simulink model "MotorXploer"  (R2024b)
settings: Solver=FixedStepAuto  StartTime=0.0  StopTime=inf  FixedStep=0.001  RelTol=1e-3
undefined symbols (not defined in the file or in its folder): Blocking, LF, Non
libraries: hdlsllib x5, amg_usbconverter_n_connect_lib x3
settings Model: Creator=beamk  LastModifiedBy=VICTUS

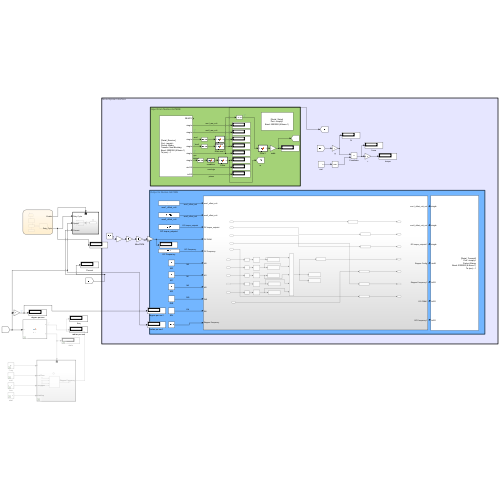
[thumbnail: Simulink's stored preview of the top-level diagram]
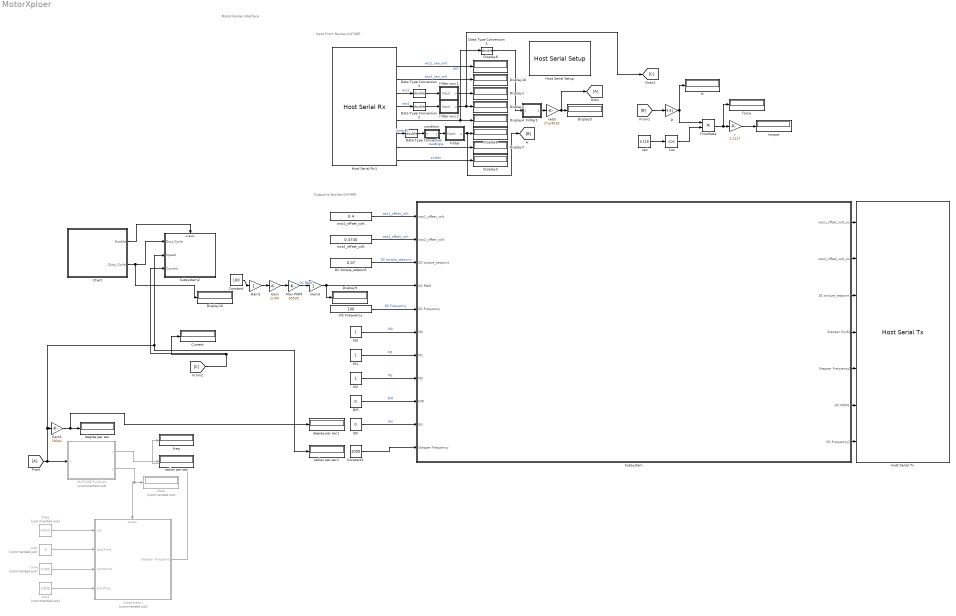
== system MotorXploer ==
  note: Output to Nucleo-G474RE
  note: Input From Nucleo-G474RE
  note: MotorXploler Interface
  Chart : Stateflow chart  TreatAsAtomicUnit=on
      settings: PortSchema="{\"entries\":[{\"content\":{\"sides\":[{\"content\":{},\"type\":\"ConnectorPlacement.EquallySpacedRectSide\",\"uuid\":\"8e28883a-1281-4b20-80f5-117cf80ab28d\"},{\"content\":{\"connectorIds\":[\"Out2\",\"Out1\"],\"side\":\"RIGHT\"},\"type\":\"ConnectorPlacement.EquallySpacedRectSide\",\"uuid\":\"8e6f6195-e9fb-4b08-ac17-6c9691bed55c\"},{\"content\":{\"side\":\"TOP\"},\"type\":\"ConnectorPlacement.EquallySpacedRectSide\",\"uuid\":\"2bfcf31e-5df8-4905-a340-c34624cfbeee\"}]},\"type\":\"ConnectorPlacement.EquallySpacedConnector\",\"uuid\":\"f3782a18-4493-4071-a1dd-9ffba4b12391\"}],\"packageUris\":[\"http://schema.mathworks.com/mf0/Connector/R2020b\"],\"version\":\"1.0\"}"
  Constant : Constant  Value=100
  Constant1 : Constant  Value=1000
  Cos : Trigonometry  Operator=cos
  Current : Display
  DC Frequency : Constant  Value=100
  DC torque_setpoint : Constant  Value=0.07
  DIR : Constant  Value=0  OutDataTypeStr=uint8
  Data Type Conversion{,1..3} (4 alike) : DataTypeConversion  OutDataTypeStr=double  SaturateOnIntegerOverflow=off  RndMeth=Floor
  Display{1..10,16} (11 alike) : Display
  EN : Constant  Value=0  OutDataTypeStr=uint8
  Fcostheta : Product
  Fillter : MATLAB Function  TreatAsAtomicUnit=on
  Fillter1 : MATLAB Function  TreatAsAtomicUnit=on
  Freq : Constant  Commented=on  Value=200000
  From : From
  Gain : Gain  Gain=1/100
  Gain1 : Gain  Gain=180/pi
  Gain2 : Gain
  Gain3 : Gain
  Goto : Goto
  Host Serial Rx1 : amg_usbconverter_n_connect_lib/Host Serial Rx  conf=rx  port=<auto>  baudrate=2000000  databits=8  parity=None  stopbit=1  flowcontrol=None  transfer=Non-Blocking  timeout=5  packetmode=Binary  enableinitialvalues=off  initialvalues=[]  binheader='45'  binterminator='A'  porttype_double=0  porttype_single=6  porttype_int8=0  porttype_uint8=0  porttype_int16=0  porttype_uint16=1  porttype_int32=1  porttype_uint32=0  asciiformat='%f,%f,%d,%d'  rx_asciiterminator="LF (0x0A - \"\\n\")"  tx_asciiterminator="CRLF (0x0D 0x0A - \"\\r\\n\")"  sampletime=-1  enablecustomportlabel=off  cinputportlabel=0  coutputportlabel=A  portpinstr=0  blockid=HostSerialRx1  inputporttype=[]  inputportwidth=[]  inputportlabel={}  outputporttype=[3 1 1 1 1 1 1 5 6]  outputportwidth=[1 1 1 1 1 1 1 1 1]  outputportlabel={'READY','single','single','single','single','single','single','uint16','int32'}  compat=0  optionstring=[]  autoport='<empty>'
  Host Serial Setup : amg_usbconverter_n_connect_lib/Host Serial Setup  conf=setup  port=<auto>  baudrate=2000000  databits=8  parity=None  stopbit=1  flowcontrol=None  transfer=Blocking  timeout=2  packetmode=Binary  initialvalues=[]  binheader='7E 7E'  binterminator='03 03'  porttype_double=0  porttype_single=1  porttype_int8=0  porttype_uint8=0  porttype_int16=0  porttype_uint16=0  porttype_int32=0  porttype_uint32=2  asciiformat='%d %u %x'  rx_asciiterminator="CRLF (0x0D 0x0A - \"\\r\\n\")"  tx_asciiterminator="CRLF (0x0D 0x0A - \"\\r\\n\")"  sampletime=-1  enablecustomportlabel=off  cinputportlabel=0  coutputportlabel=A  portpinstr=0  blockid=HostSerialSetup  inputporttype=[]  inputportwidth=[]  inputportlabel={}  outputporttype=[]  outputportwidth=[]  outputportlabel={}  compat=0  optionstring=[]  autoport='<empty>'
  Host Serial Tx : amg_usbconverter_n_connect_lib/Host Serial Tx  conf=tx  port=<auto>  baudrate=2000000  databits=8  parity=None  stopbit=1  flowcontrol=None  transfer=Blocking  timeout=2  packetmode=Binary  initialvalues=[]  binheader='45'  binterminator='A'  porttype_double=0  porttype_single=3  porttype_int8=0  porttype_uint8=1  porttype_int16=0  porttype_uint16=0  porttype_int32=3  porttype_uint32=0  asciiformat='%d,%f'  rx_asciiterminator="CRLF (0x0D 0x0A - \"\\r\\n\")"  tx_asciiterminator="CRLF (0x0D 0x0A - \"\\r\\n\")"  sampletime=-1  enablecustomportlabel=off  cinputportlabel=0  coutputportlabel=A  portpinstr=0  blockid=HostSerialTx  inputporttype=[1 1 1 3 6 6 6]  inputportwidth=[1 1 1 1 1 1 1]  inputportlabel={'single','single','single','uint8','int32','int32','int32'}  outputporttype=[]  outputportwidth=[]  outputportlabel={}  compat=0  optionstring=[]  autoport='<empty>'
      settings: SourceProductName=aMG USB Converter N
  M0 : Constant  OutDataTypeStr=uint8
  M1 : Constant  OutDataTypeStr=uint8
  M2 : Constant  OutDataTypeStr=uint8
  MATLAB Function : MATLAB Function  Commented=on  TreatAsAtomicUnit=on
  Max PWM : Gain  Gain=65535
  N : Display
  Subsystem : Subsystem
  Subsystem1 : Subsystem  Commented=on
  Subsystem2 : Subsystem
  condition : MATLAB Function  TreatAsAtomicUnit=on
  degree per sec : Display
      settings: Format=decimal (Stored Integer)
  degree per sec1 : Display
      settings: Format=decimal (Stored Integer)
  fillter wcs 1 : MATLAB Function  TreatAsAtomicUnit=on
  fillter wcs 2 : MATLAB Function  TreatAsAtomicUnit=on
  force : Display
  freq : Display
      settings: Format=decimal (Stored Integer)
  g : Gain  Gain=9.81
  r : Gain  Gain=0.1127
  rad : Constant  Value=0.118
  rad/s : Gain  Gain=2*pi/8192
  radian per sec : Display
  radian per sec1 : Display
  start : Constant  Commented=on  Value=1000
  state : Display  Commented=on
  time : Constant  Commented=on  Value=0.003
  torque : Display
  wait : Constant  Commented=on  Value=3
  wcs1_offset_volt : Constant  Value=0.4  OutDataTypeStr=single
  wcs2_offset_volt : Constant  Value=0.4745  OutDataTypeStr=single
  wires:
  Host Serial Rx1/2 -> Display8/1  "wcs1_raw_volt"
  Host Serial Rx1/3 -> Display16/1  "wcs2_raw_volt"
  Host Serial Rx1/7 -> Data Type Conversion/1  "loadcell"
  Host Serial Rx1/5 -> Data Type Conversion2/1  "wcs2"
  Host Serial Rx1/8 -> Display7/1  "rawAngle"
  rad/s/1 -> Goto/1, Display5/1
  Host Serial Rx1/6 -> Data Type Conversion1/1, Display4/1  "pps"
  Host Serial Rx1/4 -> Data Type Conversion3/1  "wcs1"
  Host Serial Rx1/9 -> Display3/1  "pulses"
  wcs1_offset_volt/1 -> Subsystem/1(wcs1_offset_volt)  "wcs1_offset_volt"
  wcs2_offset_volt/1 -> Subsystem/2(wcs2_offset_volt)  "wcs2_offset_volt"
  DC torque_setpoint/1 -> Subsystem/3(DC torque_setpoint)  "DC torque_setpoint"
  Max PWM/1 -> Gain3/1  "DC PWM"
  DC Frequency/1 -> Subsystem/5(DC Frequency)  "DC Frequency"
  M0/1 -> Subsystem/6(M0)  "M0"
  M1/1 -> Subsystem/7(M1)  "M1"
  M2/1 -> Subsystem/8(M2)  "M2"
  DIR/1 -> Subsystem/9(DIR)  "DIR"
  EN/1 -> Subsystem/10(EN)  "EN"
  Subsystem/1(wcs1_offset_volt_out) -> Host Serial Tx/1
  Subsystem/2(wcs2_offset_volt_out) -> Host Serial Tx/2
  Subsystem/3(DC torque_setpoint1) -> Host Serial Tx/3
  Subsystem/4(Stepper Config) -> Host Serial Tx/4
  Subsystem/5(Stepper Frequency1) -> Host Serial Tx/5
  Subsystem/6(DC PWM1) -> Host Serial Tx/6
  Subsystem/7(DC Frequency1) -> Host Serial Tx/7
  Fillter1/1(Output) -> rad/s/1
  Data Type Conversion1/1 -> Fillter1/1(Input)
  Subsystem1/1(Stepper Frequency) -> freq/1
  Freq/1 -> Subsystem1/1(In1)
  wait/1 -> Subsystem1/2(waitTime)
  time/1 -> Subsystem1/3(ramptime)
  start/1 -> Subsystem1/4(startfreq)
  From/1 -> Subsystem2/2(Speed), radian per sec1/1, Gain1/1, MATLAB Function/1(u)
  MATLAB Function/2(y) -> state/1, Subsystem1/Enable
  Gain1/1 -> degree per sec1/1, degree per sec/1
  MATLAB Function/1(x) -> radian per sec/1
  Data Type Conversion/1 -> condition/1(u)
  condition/1(y) -> Fillter/1(Input)
  Fillter/1(u) -> [B], Display6/1
  [B] -> g/1
  g/1 -> N/1, Fcostheta/1
  rad/1 -> Cos/1
  Cos/1 -> Fcostheta/2
  Fcostheta/1 -> force/1, r/1
  r/1 -> torque/1
  fillter wcs 2/1(u) -> [C], Display2/1
  Data Type Conversion2/1 -> fillter wcs 2/1(Input)
  Data Type Conversion3/1 -> fillter wcs 1/1(Input)
  fillter wcs 1/1(u) -> Display1/1
  Gain/1 -> Max PWM/1
  [C] -> Subsystem2/3(Current), Current/1
  Gain2/1 -> Gain/1
  Gain3/1 -> Display9/1, Subsystem/4(DC PWM)
  Chart/1(Duty_Cycle) -> Display10/1, Subsystem2/1(Duty Cycle)
  Chart/2(Enable) -> Subsystem2/Enable
  Constant/1 -> Gain2/1
  Constant1/1 -> Subsystem/11(Stepper Frequency)

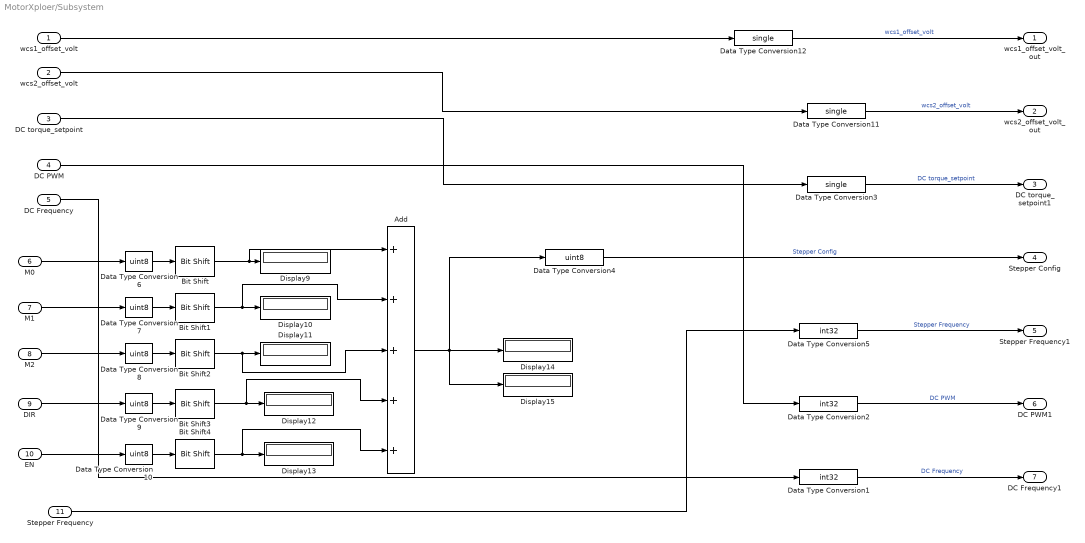
== system MotorXploer/Subsystem ==
  wcs1_offset_volt : Inport
  wcs2_offset_volt : Inport  Port=2
  DC torque_setpoint : Inport  Port=3
  DC PWM : Inport  Port=4
  DC Frequency : Inport  Port=5
  M0 : Inport  Port=6
  M1 : Inport  Port=7
  M2 : Inport  Port=8
  DIR : Inport  Port=9
  EN : Inport  Port=10
  Stepper Frequency : Inport  Port=11
  Add : Sum  Inputs=+++++
  Bit Shift : hdlsllib/Logic and Bit Operations/Bit Shift  mode=Shift Left Logical  N=4
  Bit Shift1 : hdlsllib/Logic and Bit Operations/Bit Shift  mode=Shift Left Logical  N=3
  Bit Shift2 : hdlsllib/Logic and Bit Operations/Bit Shift  mode=Shift Left Logical  N=2
  Bit Shift3 : hdlsllib/Logic and Bit Operations/Bit Shift  mode=Shift Left Logical  N=1
  Bit Shift4 : hdlsllib/Logic and Bit Operations/Bit Shift  mode=Shift Left Logical  N=0
  Data Type Conversion1 : DataTypeConversion  OutDataTypeStr=int32  SaturateOnIntegerOverflow=off  RndMeth=Floor
  Data Type Conversion{4,6..10} (6 alike) : DataTypeConversion  OutDataTypeStr=uint8  SaturateOnIntegerOverflow=off  RndMeth=Floor
  Data Type Conversion11 : DataTypeConversion  OutDataTypeStr=single  SaturateOnIntegerOverflow=off  RndMeth=Floor
  Data Type Conversion12 : DataTypeConversion  OutDataTypeStr=single  SaturateOnIntegerOverflow=off  RndMeth=Floor
  Data Type Conversion2 : DataTypeConversion  OutDataTypeStr=int32  SaturateOnIntegerOverflow=off  RndMeth=Floor
  Data Type Conversion3 : DataTypeConversion  OutDataTypeStr=single  SaturateOnIntegerOverflow=off  RndMeth=Floor
  Data Type Conversion5 : DataTypeConversion  OutDataTypeStr=int32  SaturateOnIntegerOverflow=off  RndMeth=Floor
  Display{9..15} (7 alike) : Display
      Display10 settings: Format=binary (Stored Integer)
      Display11 settings: Format=binary (Stored Integer)
      Display12 settings: Format=binary (Stored Integer)
      Display13 settings: Format=binary (Stored Integer)
      Display14 settings: Format=binary (Stored Integer)
      Display9 settings: Format=binary (Stored Integer)
  wcs1_offset_volt_out : Outport
  wcs2_offset_volt_out : Outport  Port=2
  DC torque_setpoint1 : Outport  Port=3
  Stepper Config : Outport  Port=4
  Stepper Frequency1 : Outport  Port=5
  DC PWM1 : Outport  Port=6
  DC Frequency1 : Outport  Port=7
  wires:
  Bit Shift/1 -> Display9/1, Add/1
  Data Type Conversion8/1 -> Bit Shift2/1
  EN/1 -> Data Type Conversion10/1
  Data Type Conversion6/1 -> Bit Shift/1
  DC torque_setpoint/1 -> Data Type Conversion3/1
  Data Type Conversion2/1 -> DC PWM1/1  "DC PWM"
  Data Type Conversion7/1 -> Bit Shift1/1
  Data Type Conversion10/1 -> Bit Shift4/1
  DC PWM/1 -> Data Type Conversion2/1
  Bit Shift3/1 -> Display12/1, Add/4
  Data Type Conversion12/1 -> wcs1_offset_volt_out/1  "wcs1_offset_volt"
  Add/1 -> Display15/1, Display14/1, Data Type Conversion4/1
  Bit Shift2/1 -> Display11/1, Add/3
  Stepper Frequency/1 -> Data Type Conversion5/1
  M1/1 -> Data Type Conversion7/1
  Bit Shift1/1 -> Display10/1, Add/2
  Bit Shift4/1 -> Display13/1, Add/5
  M0/1 -> Data Type Conversion6/1
  Data Type Conversion9/1 -> Bit Shift3/1
  Data Type Conversion11/1 -> wcs2_offset_volt_out/1  "wcs2_offset_volt"
  M2/1 -> Data Type Conversion8/1
  wcs1_offset_volt/1 -> Data Type Conversion12/1
  DC Frequency/1 -> Data Type Conversion1/1
  wcs2_offset_volt/1 -> Data Type Conversion11/1
  Data Type Conversion1/1 -> DC Frequency1/1  "DC Frequency"
  DIR/1 -> Data Type Conversion9/1
  Data Type Conversion4/1 -> Stepper Config/1  "Stepper Config"
  Data Type Conversion3/1 -> DC torque_setpoint1/1  "DC torque_setpoint"
  Data Type Conversion5/1 -> Stepper Frequency1/1  "Stepper Frequency"

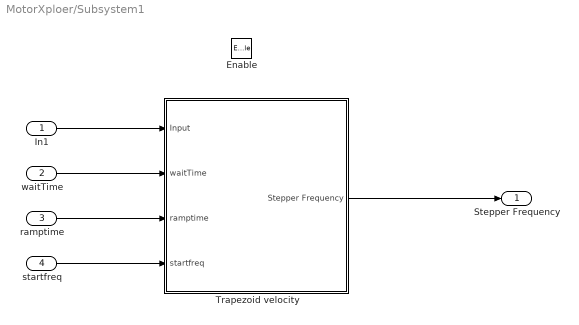
== system MotorXploer/Subsystem1 ==
  In1 : Inport
  waitTime : Inport  Port=2
  ramptime : Inport  Port=3
  startfreq : Inport  Port=4
  Enable : EnablePort
  Trapezoid velocity : MATLAB Function  TreatAsAtomicUnit=on
  Stepper Frequency : Outport
  wires:
  In1/1 -> Trapezoid velocity/1(Input)
  Trapezoid velocity/1(Stepper Frequency) -> Stepper Frequency/1
  startfreq/1 -> Trapezoid velocity/4(startfreq)
  waitTime/1 -> Trapezoid velocity/2(waitTime)
  ramptime/1 -> Trapezoid velocity/3(ramptime)

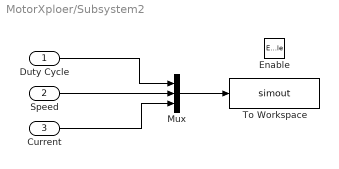
== system MotorXploer/Subsystem2 ==
  Duty Cycle : Inport
  Speed : Inport  Port=2
  Current : Inport  Port=3
  Enable : EnablePort
  Mux : Mux  Inputs=3
  To Workspace : ToWorkspace  VariableName=simout  SampleTime=-1
  wires:
  Duty Cycle/1 -> Mux/1
  Speed/1 -> Mux/2
  Current/1 -> Mux/3
  Mux/1 -> To Workspace/1

== matlab function MotorXploer/Fillter1 ==
  data: Input input; Output output
function Output = fcn(Input)
    persistent Buffer
    persistent first
    persistent last
    persistent curr
    persistent tmp

    if isempty(Buffer)
        Buffer = [];
        first = 1;
        last = 1125;
        curr = 0;
        tmp = Input;
    end

    Buffer(end+1) = Input;

    if curr >= last
        first = first + 1;
        last = last + 1;
        tmp = mean(Buffer(first:last));
    end

    curr = curr + 1;
    Output = tmp;

end

== matlab function MotorXploer/Fillter ==
  data: Input input; Output output
function Output = fcn(Input)
    persistent Buffer
    persistent first
    persistent last
    persistent curr
    persistent tmp

    if isempty(Buffer)
        Buffer = [];
        first = 1;
        last = 1000;
        curr = 0;
        tmp = Input;
    end

    Buffer(end+1) = Input;

    if curr >= last
        first = first + 1;
        last = last + 1;
        tmp = mean(Buffer(first:last));
    end

    curr = curr + 1;
    Output = tmp;

end

== matlab function MotorXploer/Subsystem1/Trapezoid velocity ==
  data: Input input; Output output; waitTime input; ramptime input; startfreq input
function Output = fcn(Input,waitTime,ramptime,startfreq)

    persistent freq
    persistent time
    persistent mode
    persistent prev

    if isempty(freq)
        freq = 0;
        time = 0;
        mode = 0;
        prev = 0;
    end

    if mode == 0
        if time >= 0.1
            freq = freq + (startfreq * 0.05);
            time = 0;
            if freq == startfreq
                mode = 2;
                time = 0;
                prev = freq;
            end
        end
    elseif mode == 1
        if time >= ramptime && freq < Input && (freq < 17000 || freq > 17999)
            freq = freq + 0.5;
            time = 0;
            if freq - prev == 1000.0
                prev = freq;
                mode = 2;
                time = 0;
            end
        elseif time >= ramptime && freq < Input && (freq >= 17000 && freq <= 17999)
            freq = freq + 500;
            time = 0;
            if freq - prev == 1000.0
                prev = freq;
                mode = 2;
                time = 0;
            end
        end
    else
        if time >= waitTime
            mode = 1;
            time = 0;
        end
    end

    time = time + 0.001;

    Output = freq;


end

== matlab function MotorXploer/MATLAB Function ==
  data: x output; u input; y output
function [x,y] = fcn(u)
    persistent prev
    persistent state
    persistent max

    if isempty(prev)
        prev = u*0.8;
        state = 1;
        max = prev/0.8;
    end

    if abs(u) < abs(prev)
        state = 0;
        
    end

    if abs(max) < abs(prev/0.8)
        max = prev/0.8;
    end

    x = max;
    prev = u*0.8;
    y = state;
        

end

== matlab function MotorXploer/condition ==
  data: u input; y output
function y = fcn(u)
    y = ((-7 * power(10,-22)) * power(u,6)) + ((1 * power(10,-16)) * power(u,5)) - ((7 * power(10,-13)) * power(u,4)) + ((2 * power(10,-9)) * power(u,3)) - ((3 * power(10,-6)) * power(u,2)) + (0.0027 * u) - 0.2084;
end

== matlab function MotorXploer/fillter wcs 2 ==
  data: Input input; Output output
function Output = fcn(Input)
    persistent Buffer
    persistent first
    persistent last
    persistent curr
    persistent tmp

    if isempty(Buffer)
        Buffer = [];
        first = 1;
        last = 750;
        curr = 0;
        tmp = Input;
    end

    Buffer(end+1) = Input;

    if curr >= last
        first = first + 1;
        last = last + 1;
        tmp = mean(Buffer(first:last));
    end

    curr = curr + 1;
    Output = tmp;

end

== matlab function MotorXploer/fillter wcs 1 ==
  data: Input input; Output output
function Output = fcn(Input)
    persistent Buffer
    persistent first
    persistent last
    persistent curr
    persistent tmp

    if isempty(Buffer)
        Buffer = [];
        first = 1;
        last = 750;
        curr = 0;
        tmp = Input;
    end

    Buffer(end+1) = Input;

    if curr >= last
        first = first + 1;
        last = last + 1;
        tmp = mean(Buffer(first:last));
    end

    curr = curr + 1;
    Output = tmp;

end

== stateflow chart MotorXploer/Chart ==
  state init
    time = 0;
    Enable = 0;
    Duty_Cycle = 0;
  state first_step
    entry:
    Enable = 1;
    exit:
    Enable = 0;
    Duty_Cycle = 1;
  state Active
    entry:
    Enable = 1;
    exit:
    Enable = 0;
    Duty_Cycle = Duty_Cycle + 1;
    time = 0;
  state wait
    during:
    time = time + 0.001;
  state Stop
    Duty_Cycle = 0;
  (default) -> init
  init -> first_step
  first_step -> wait
  Active -> wait
  wait -> Active [order 1] : [time >= 3.000]
  wait -> Stop [order 2] : [Duty_Cycle > 100]
  data: time local; Duty_Cycle output; Enable output
